simulink model "Simulink_PLC_coder_example"  (R2022a)
settings: Solver=FixedStepDiscrete  StartTime=0.0  StopTime=10  FixedStep=0.0001  RelTol=1e-3
values from neighbouring files (symbols this model uses):
  tCycle = 0.001    [param.m]
settings Model: Creator=Jan Størbu  LastModifiedBy=endre
settings SolverCC: AlgebraicLoopSolver=TrustRegion
settings DataIOCC: ReturnWorkspaceOutputs=off
settings DebuggingCC: UnconnectedInputMsg=warning  UnconnectedOutputMsg=warning  UnconnectedLineMsg=warning  BusObjectLabelMismatch=error  SFMachineParentedDataDiag=warning  ArithmeticOperatorsInVariantConditions=warning
settings SFSimCC: SimUseLocalCustomCode=off  CustomCodeUndefinedFunction=UseInterfaceOnly
settings RTWCC: RTWUseLocalCustomCode=off  DLArmComputeVersion=19.05
settings ConfigComp: PLC_TargetIDE=plcopen  PLC_MultiTBSigbuilderTimeRange=off  PLC_ReuseMLFcnVariable=on  PLC_InlineEnumCastFunction=off  PLC_GenerateReport=off  PLC_LaunchReport=off

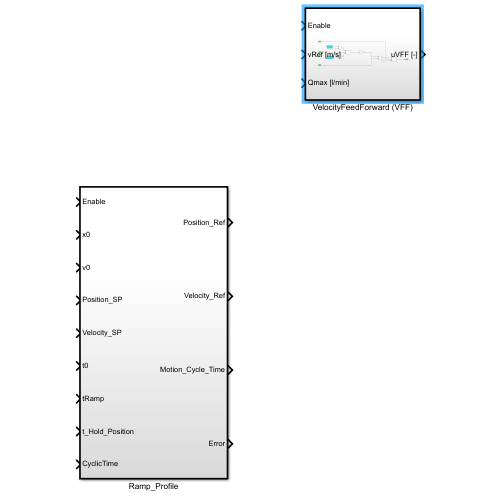
[thumbnail: Simulink's stored preview of the top-level diagram]
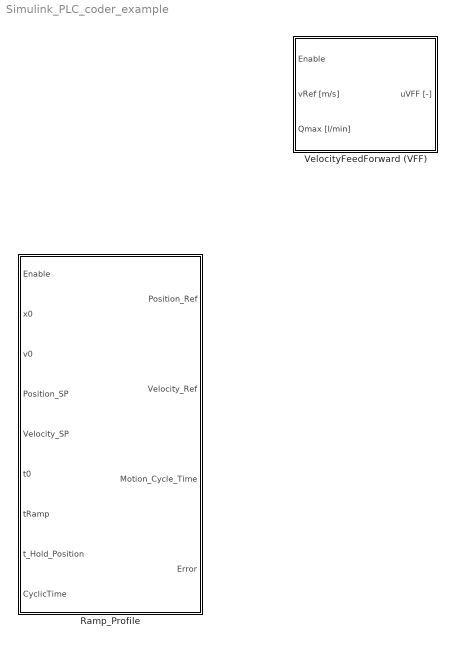
== system Simulink_PLC_coder_example ==
  Ramp_Profile : Subsystem  TreatAsAtomicUnit=on  VariantControl=Ramp_Profile
  VelocityFeedForward (VFF) : Subsystem  TreatAsAtomicUnit=on  SystemSampleTime=tCycle

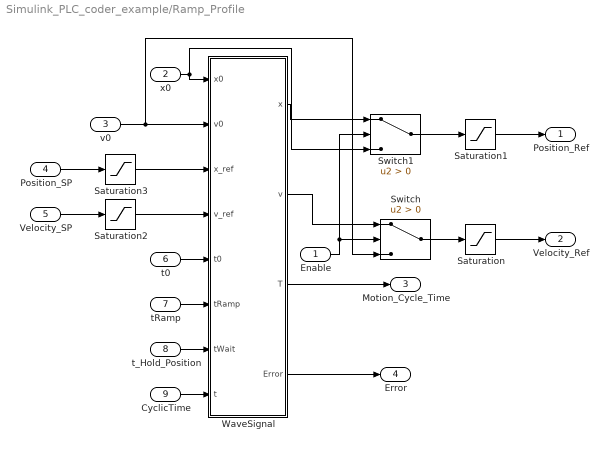
== system Simulink_PLC_coder_example/Ramp_Profile ==
  Enable : Inport  OutDataTypeStr=boolean
  x0 : Inport  Port=2
  v0 : Inport  Port=3
  Position_SP : Inport  Port=4
  Velocity_SP : Inport  Port=5
  t0 : Inport  Port=6
  tRamp : Inport  Port=7
  t_Hold_Position : Inport  Port=8
  CyclicTime : Inport  Port=9
  Saturation : Saturate  UpperLimit=150  LowerLimit=-150
  Saturation1 : Saturate  UpperLimit=500  LowerLimit=0
  Saturation2 : Saturate  UpperLimit=150  LowerLimit=0
  Saturation3 : Saturate  UpperLimit=500  LowerLimit=0
  Switch : Switch  Criteria=u2 > Threshold  SaturateOnIntegerOverflow=off  InputSameDT=off
  Switch1 : Switch  Criteria=u2 > Threshold  SaturateOnIntegerOverflow=off  InputSameDT=off
  WaveSignal : MATLAB Function  TreatAsAtomicUnit=on
  Position_Ref : Outport  VectorParamsAs1DForOutWhenUnconnected=off
  Velocity_Ref : Outport  Port=2  VectorParamsAs1DForOutWhenUnconnected=off
  Motion_Cycle_Time : Outport  Port=3  VectorParamsAs1DForOutWhenUnconnected=off
  Error : Outport  Port=4  VectorParamsAs1DForOutWhenUnconnected=off
  wires:
  CyclicTime/1 -> WaveSignal/8(t)
  WaveSignal/2(v) -> Switch/1
  Switch/1 -> Saturation/1
  v0/1 -> Switch/3, WaveSignal/2(v0)
  t0/1 -> WaveSignal/5(t0)
  Position_SP/1 -> Saturation3/1
  t_Hold_Position/1 -> WaveSignal/7(tWait)
  Velocity_SP/1 -> Saturation2/1
  WaveSignal/1(x) -> Switch1/1
  WaveSignal/3(T) -> Motion_Cycle_Time/1
  Enable/1 -> Switch1/2, Switch/2
  x0/1 -> Switch1/3, WaveSignal/1(x0)
  Switch1/1 -> Saturation1/1
  Saturation/1 -> Velocity_Ref/1
  Saturation1/1 -> Position_Ref/1
  WaveSignal/4(Error) -> Error/1
  Saturation2/1 -> WaveSignal/4(v_ref)
  Saturation3/1 -> WaveSignal/3(x_ref)
  tRamp/1 -> WaveSignal/6(tRamp)

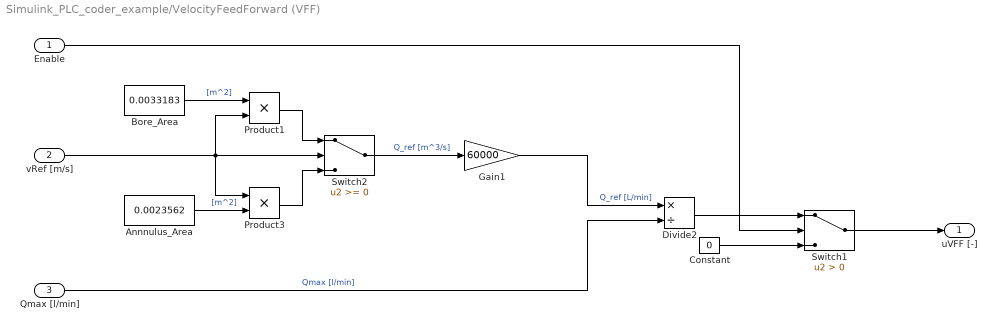
== system Simulink_PLC_coder_example/VelocityFeedForward (VFF) ==
  Enable : Inport  OutDataTypeStr=boolean
  vRef [m/s] : Inport  Port=2
  Qmax [l/min] : Inport  Port=3
  Annnulus_Area : Constant  Value=0.0023562
  Bore_Area : Constant  Value=0.0033183
  Constant : Constant  Value=0
  Divide2 : Product  Inputs=*/
  Gain1 : Gain  Gain=60000
  Product1 : Product
  Product3 : Product
  Switch1 : Switch  Criteria=u2 > Threshold  SaturateOnIntegerOverflow=off  InputSameDT=off
  Switch2 : Switch  SaturateOnIntegerOverflow=off  InputSameDT=off
  uVFF [-] : Outport  VectorParamsAs1DForOutWhenUnconnected=off
  wires:
  Annnulus_Area/1 -> Product3/2  "[m^2]"
  Switch2/1 -> Gain1/1  "Q_ref [m^3/s]"
  Product1/1 -> Switch2/1
  vRef [m/s]/1 -> Product3/1, Product1/2, Switch2/2
  Qmax [l/min]/1 -> Divide2/2  "Qmax [l/min]"
  Bore_Area/1 -> Product1/1  "[m^2]"
  Gain1/1 -> Divide2/1  "Q_ref [L/min]"
  Product3/1 -> Switch2/3
  Constant/1 -> Switch1/3
  Divide2/1 -> Switch1/1
  Enable/1 -> Switch1/2
  Switch1/1 -> uVFF [-]/1

== matlab function Simulink_PLC_coder_example/Ramp_Profile/WaveSignal ==
  data: x0 input; v0 input; x_ref input; x output; v_ref input; t0 input; tRamp input; tWait input; v output; t input; T output; Error output
function [x,v,T, Error] = fcn(x0,v0, x_ref,v_ref,t0,tRamp,tWait,t)
x_SP = x_ref - x0;
vs=v_ref;
slopeExt=v0-vs;
slopeRetr=-vs-v0;

as = vs/tRamp;
s_acc=(vs^2-v0^2)/as;

tHold=(x_SP-s_acc)/vs;

if tHold < 0 
Error = 1;
else 
Error = 0;
end

t1=tRamp;
t2=tHold; 
t3=tRamp;
t4=tWait;
t5=t1;
t6=t2;
t7=t3;

x = x0;
x1 = x0 + v0*((t0+t1)-t0)-(slopeExt/t1)*((t0+t1)-t0)^2/2;
x2 = x1 + vs*((t0+t1+t2)-(t0+t1)); 
x4 = x_ref - v0*((t0+t1+t2+t3+t4+t5)-(t0+t1+t2+t3+t4))+(slopeRetr/t5)*((t0+t1+t2+t3+t4+t5)-(t0+t1+t2+t3+t4))^2/2; 
x5 = x4-vs*((t0+t1+t2+t3+t4+t5+t6)-(t0+t1+t2+t3+t4+t5));  

if Error == 1
x = x0;
v = v0; 
elseif t>=0 && t<t0
x = x0; 
v = v0;
elseif t>=t0 && t<(t0+t1)
x = x0 + v0*(t-t0)-(slopeExt/t1)*(t-t0)^2/2;
v = v0-(slopeExt/t1)*(t-t0);  
elseif t>=(t0+t1) && t<(t0+t1+t2)
x = x1 + vs*(t-(t0+t1)); 
v = vs; 
elseif t>=(t0+t1+t2) && t<(t0+t1+t2+t3)
x = x2+vs*(t-(t0+t1+t2))+(slopeExt/t3)*(t-(t0+t1+t2))^2/2; 
v = vs+(slopeExt/t3)*(t-(t0+t1+t2));   
elseif t>=(t0+t1+t2+t3) && t<(t0+t1+t2+t3+t4)
x = x_ref;
v = v0;  
elseif t>=(t0+t1+t2+t3+t4) && t<(t0+t1+t2+t3+t4+t5)
x = x_ref - v0*(t-(t0+t1+t2+t3+t4))+(slopeRetr/t5)*(t-(t0+t1+t2+t3+t4))^2/2; 
v = v0+(slopeRetr/t5)*(t-(t0+t1+t2+t3+t4));     
elseif t>=(t0+t1+t2+t3+t4+t5) && t<(t0+t1+t2+t3+t4+t5+t6)
x = x4-vs*(t-(t0+t1+t2+t3+t4+t5));   
v = -vs;    
elseif t>=(t0+t1+t2+t3+t4+t5+t6) && t<(t0+t1+t2+t3+t4+t5+t6+t7)
x = x5-vs*(t-(t0+t1+t2+t3+t4+t5+t6))-(slopeRetr/t3)*(t-(t0+t1+t2+t3+t4+t5+t6))^2/2;    
v = -vs-(slopeRetr/t3)*(t-(t0+t1+t2+t3+t4+t5+t6));     
else 
x = x0;
v = v0; 
end

T = t0+t1+t2+t3+t4+t5+t6+t7;
